simulink model "interp_compare_fixedpoint_R2019a"  (R2019a)
settings: Solver=FixedStepDiscrete  StartTime=0.0  StopTime=1  FixedStep=1  RelTol=1e-3
Description:
  | 2-D fixed-point Lagrange vs point-slope
settings Model: Creator=Administrator  LastModifiedBy=Administrator
settings DebuggingCC: UnconnectedInputMsg=none  UnconnectedOutputMsg=none  UnconnectedLineMsg=none
settings ModelReferenceCC: UpdateModelReferenceTargets=IfOutOfDate  EnableRefExpFcnMdlSchedulingChecks=off
settings RTWCC: Description=Generic Real-Time Target
settings ConfigComp: CovBoundaryAbsTol=1.0e-5

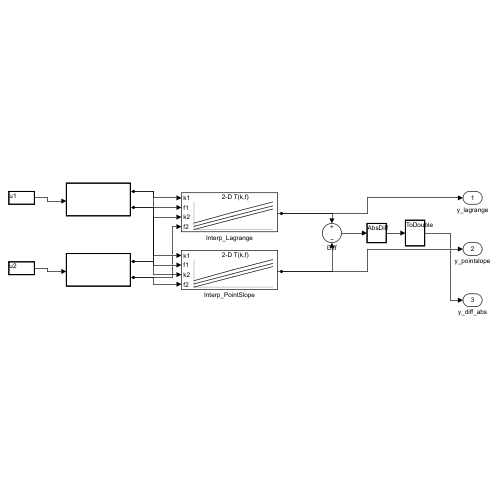
[thumbnail: Simulink's stored preview of the top-level diagram]
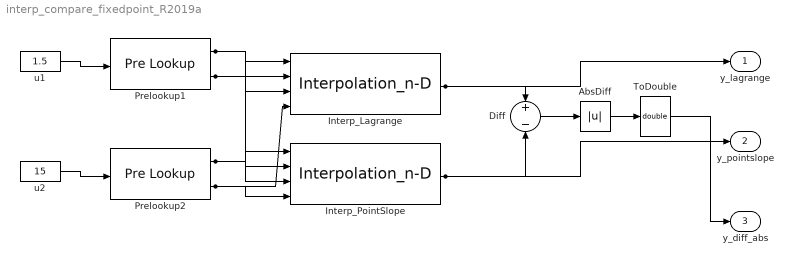
== system interp_compare_fixedpoint_R2019a ==
  AbsDiff : Abs
  Diff : Sum  Inputs=+-
  Interp_Lagrange : Interpolation_n-D  Table=[100 200 300;400 500 600;700 800 900]  InterpMethod=Linear Lagrange  ExtrapMethod=Clip  OutDataTypeStr=fixdt(1,16,4)  InternalRulePriority=Speed  TableDataTypeStr=fixdt(1,16,4)
  Interp_PointSlope : Interpolation_n-D  Table=[100 200 300;400 500 600;700 800 900]  ExtrapMethod=Clip  OutDataTypeStr=fixdt(1,16,4)  InternalRulePriority=Speed  TableDataTypeStr=fixdt(1,16,4)
  Prelookup1 : PreLookup  BreakpointsData=[1 2 3]  IndexDataTypeStr=uint16  FractionDataTypeStr=fixdt(1,16,8)
  Prelookup2 : PreLookup  BreakpointsData=[10 20 30]  IndexDataTypeStr=uint16  FractionDataTypeStr=fixdt(1,16,8)
  ToDouble : DataTypeConversion  OutDataTypeStr=double
  u1 : Constant  Value=1.5  OutDataTypeStr=double
  u2 : Constant  Value=15  OutDataTypeStr=double
  y_lagrange : Outport
  y_pointslope : Outport  Port=2
  y_diff_abs : Outport  Port=3
  wires:
  u1/1 -> Prelookup1/1
  u2/1 -> Prelookup2/1
  Prelookup1/1 -> Interp_Lagrange/1, Interp_PointSlope/1
  Prelookup1/2 -> Interp_Lagrange/2, Interp_PointSlope/2
  Prelookup2/1 -> Interp_Lagrange/3, Interp_PointSlope/3
  Prelookup2/2 -> Interp_Lagrange/4, Interp_PointSlope/4
  Interp_Lagrange/1 -> Diff/1, y_lagrange/1
  Interp_PointSlope/1 -> Diff/2, y_pointslope/1
  Diff/1 -> AbsDiff/1
  AbsDiff/1 -> ToDouble/1
  ToDouble/1 -> y_diff_abs/1
